simulink model "xPC_UDP"  (R2016a)
settings: Solver=ode3  StartTime=0.0  StopTime=inf  FixedStep=dt  RelTol=1e-3
InitFcn:
  | XPCUDP_DEPENDENCY
  | init_xPC_UDP
  | init_udp
undefined symbols (not defined in the file or in its folder): dt
libraries: etargetslib x2, xpcrtudplib x2, slrtlib x1, xpcobsoletelib x1, simulink x1
settings Model: Creator=Andrea  LastModifiedBy=garrison
settings SolverCC: EnableConcurrentExecution=on
settings DataIOCC: LimitDataPoints=on  SaveFormat=Array  SignalLoggingSaveFormat=ModelDataLogs
settings OptimizationCC: BlockReduction=off  OptimizeBlockIOStorage=off  BufferReuse=off  GlobalBufferReuse=off  ExpressionFolding=off  ExpressionDepthLimit=2147483647  LocalBlockOutputs=off  OptimizeModelRefInitCode=on
settings DebuggingCC: UnderspecifiedInitializationDetection=Classic  MergeDetectMultiDrivingBlocksExec=none  SolverPrmCheckMsg=warning  MultiTaskCondExecSysMsg=warning  MultiTaskRateTransMsg=warning  FcnCallInpInsideContextMsg=UseLocalSettings  StateNameClashWarn=warning
settings HardwareCC: ProdBitPerPointer=32  ProdLargestAtomicFloat=None  ProdWordSize=32  ProdLongLongMode=on  ProdHWDeviceType=Generic->32-bit x86 compatible
settings ModelReferenceCC: PropagateSignalLabelsOutOfModel=off
settings SFSimCC: SimParseCustomCode=off
settings RTWCC: SystemTargetFile=slrtert.tlc  TemplateMakefile=slrtert_default_tmf  Description=Simulink Real-Time (ERT)  RTWCompilerOptimization=on
settings CodeAppCC: CustomSymbolStrType=$N$R$M  InternalIdentifier=Classic
settings SimulinkRealTimeERTCC: TargetFcnLib=ansi_tfl_table_tmw.mat  GenFloatMathFcnCalls=NOT IN USE  TargetLangStandard=C89/C90 (ANSI)  CodeReplacementLibrary=XPC_BLAS  UtilityFuncGeneration=Auto  ERTMultiwordTypeDef=System defined  ERTMultiwordLength=256  MultiwordLength=2048  GenerateFullHeader=on  InferredTypesCompatibility=off  GenerateSampleERTMain=off  GenerateTestInterfaces=off  ModelReferenceCompliant=on  ParMdlRefBuildCompliant=on  CompOptLevelCompliant=on  ConcurrentExecutionCompliant=on  IncludeMdlTerminateFcn=on  GeneratePreprocessorConditionals=Disable all  CombineOutputUpdateFcns=off  CombineSignalStateStructs=off  SuppressErrorStatus=off  ERTFirstTimeCompliant=off  IncludeFileDelimiter=Auto  ERTCustomFileBanners=off  SupportAbsoluteTime=on  LogVarNameModifier=rt_  MatFileLogging=on  MultiInstanceERTCode=off  CodeInterfacePackaging=Nonreusable function  SupportNonFinite=on  SupportComplex=on  PurelyIntegerCode=off  SupportContinuousTime=on  SupportNonInlinedSFcns=on  SupportVariableSizeSignals=off  ParenthesesLevel=Nominal  CastingMode=Nominal  MATLABClassNameForMDSCustomization=xpcAperiodicCustomization  ModelStepFunctionPrototypeControlCompliant=off  CPPClassGenCompliant=off  AutosarCompliant=off  GRTInterface=on  GenerateAllocFcn=off  UseToolchainInfoCompliant=off  GenerateSharedConstants=on  ExtModeTransport=0  ExtModeStaticAlloc=off  ExtModeStaticAllocSize=1000000  ExtModeTesting=off  InlinedParameterPlacement=Hierarchical  TargetOS=BareBoardExample  MultiInstanceErrorCode=Error  RateGroupingCode=on  RootIOFormat=Individual arguments  RTWCAPIRootIO=off  EnableDataOwnership=off  ERTFilePackagingFormat=Modular  PreserveExpressionOrder=off  PreserveIfCondition=off  ConvertIfToSwitch=off  PreserveExternInFcnDecls=on  SuppressUnreachableDefaultCases=off  EnableSignedLeftShifts=on  EnableSignedRightShifts=on  IndentStyle=K&R  IndentSize=2  EnableUserReplacementTypes=off  MaxIdInt32=MAX_int32_T  MinIdInt32=MIN_int32_T  MaxIdUint32=MAX_uint32_T  MaxIdInt16=MAX_int16_T  MinIdInt16=MIN_int16_T  MaxIdUint16=MAX_uint16_T  MaxIdInt8=MAX_int8_T  MinIdInt8=MIN_int8_T  MaxIdUint8=MAX_uint8_T  BooleanTrueId=true  BooleanFalseId=false  MemSecPackage=--- None ---  MemSecDataConstants=Default  MemSecDataIO=Default  MemSecDataInternal=Default  MemSecDataParameters=Default  MemSecFuncInitTerm=Default  MemSecFuncExecute=Default  MemSecFuncSharedUtil=Default  GlobalDataDefinition=Auto  GlobalDataReference=Auto  GenerateASAP2=off  ERTSrcFileBannerTemplate=ert_code_template.cgt  ERTHdrFileBannerTemplate=ert_code_template.cgt  ERTDataSrcFileTemplate=ert_code_template.cgt  ERTDataHdrFileTemplate=ert_code_template.cgt  ERTCustomFileTemplate=example_file_process.tlc  SignalDisplayLevel=10  ParamTuneLevel=10  InitialValueSource=Model  RTWCAPISignals=off  RTWCAPIParams=on  RTWCAPIStates=off  RL32ModeModifier=Real-Time  ExtMode=on  ExtModeMexFile=ext_xpc  ExtModeIntrfLevel=Level2 - Open  ExtModeArmWhenConnect=off  RL32LogTETModifier=on  RL32LogBufSizeModifier=100000  xPCTaskExecutionProfile=off  xPCRL32EventNumber=5000  RL32IRQSourceModifier=Timer  xPCIRQSourceBoard=None/Other  xPCIOIRQSlot=-1  xpcObjCom=off  xPCGenerateASAP2=off  xPCGenerateXML=off  RL32ObjectName=tg  xPCisDownloadable=off  xPCisDefaultEnv=on  xPCisModelTimeout=on  xPCModelTimeoutSecs=5  xpcDblBuff=off  xPCLoadParamSetFile=off  xPCConcurrentTasks=off  xPCEnableSFAnimation=off
settings ConfigComp: CovModelRefEnable=Off

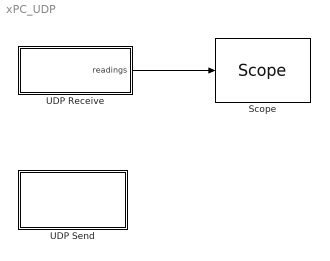
== system xPC_UDP ==
  "Scope " : slrtlib/Displays and Logging/Scope   scopeno=1  scopetype=Target  autostart=on  viewmode=Numerical  formatstr='%15.6f'  grid=on  ylimits=[0,0]  nosamples=250  noprepostsamples=0  interleave=1  triggermode=FreeRun  triggersignal=1  trigsignalfromport=off  triggerlevel=0.0  triggerslope=Either  triggerscope=1  triggersample=0  filename=data.dat  mode=Lazy  writesize=512  autorestart=off  dynamicfilemode=off  maxwritefilesize=512*1024^2
  UDP Receive : Subsystem  TreatAsAtomicUnit=on
      mask Display: %image(imread('trakSTAR.jpg'));
  UDP Send : Subsystem
  wires:
  UDP Receive/1(readings) -> "Scope "/1

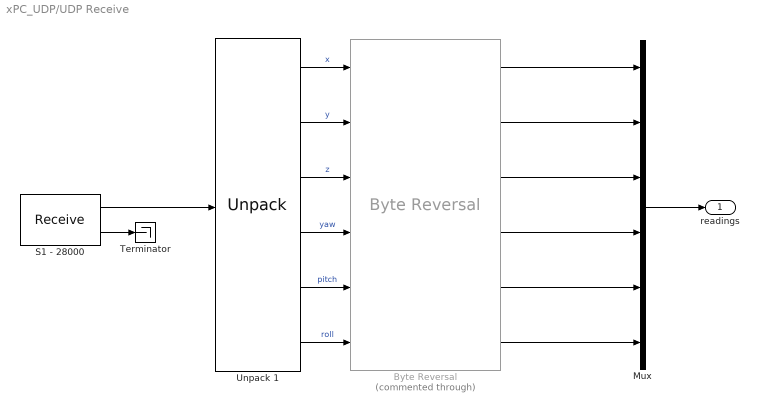
== system xPC_UDP/UDP Receive ==
  Byte Reversal : etargetslib/Byte Reversal  Commented=through  numInp=6
  Mux : Mux  Inputs=6
  S1 - 28000 : xpcrtudplib/Legacy UDP/Receive   ipAddress=0.0.0.0  ipPort=28000  width=48  vblLen=on  sampletime=dt_udp
  Terminator : Terminator
  Unpack 1 : xpcobsoletelib/Utilities/Unpack   dimensions={1,1,1,1,1,1}  datatypes={'double' 'double' 'double' 'double' 'double' 'double'}  byteAlign=1
  readings : Outport
  wires:
  S1 - 28000/1 -> Unpack 1/1
  S1 - 28000/2 -> Terminator/1
  Byte Reversal/1 -> Mux/1
  Byte Reversal/2 -> Mux/2
  Byte Reversal/3 -> Mux/3
  Byte Reversal/4 -> Mux/4
  Byte Reversal/5 -> Mux/5
  Byte Reversal/6 -> Mux/6
  Unpack 1/6 -> Byte Reversal/6  "roll"
  Unpack 1/5 -> Byte Reversal/5  "pitch"
  Unpack 1/4 -> Byte Reversal/4  "yaw"
  Unpack 1/3 -> Byte Reversal/3  "z"
  Unpack 1/2 -> Byte Reversal/2  "y"
  Unpack 1/1 -> Byte Reversal/1  "x"
  Mux/1 -> readings/1

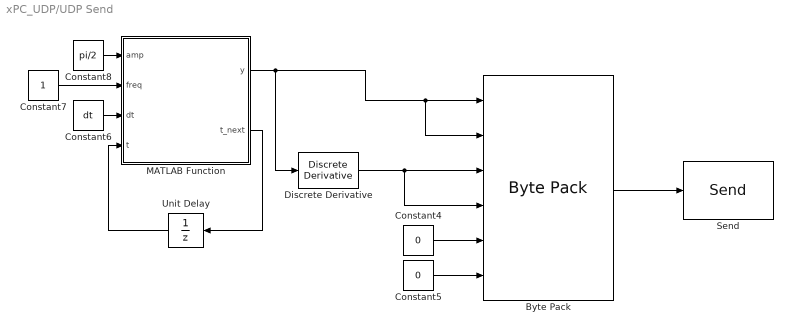
== system xPC_UDP/UDP Send ==
  Byte Pack : etargetslib/Byte Pack  datatypes={'double' 'double' 'double' 'double' 'double' 'double'}  byteAlign=1
  Constant4 : Constant  Value=0
  Constant5 : Constant  Value=0
  Constant6 : Constant  Value=dt
  Constant7 : Constant
  Constant8 : Constant  Value=pi/2
  Discrete Derivative : simulink/Discrete/Discrete Derivative  gainval=1  ICPrevScaledInput=0.0  OutMin=[]  OutMax=[]  OutDataType=fixdt(1, 16)  OutScaling=2^-10  DoSatur=off
  MATLAB Function : MATLAB Function  TreatAsAtomicUnit=on
  "Send " : xpcrtudplib/Legacy UDP/Send   ipAddress=192.168.1.30  ipPort=28001  localPort=-1  vblLen=off  sampletime=dt_udp
  Unit Delay : UnitDelay  SampleTime=-1
  wires:
  Byte Pack/1 -> "Send "/1
  Constant5/1 -> Byte Pack/6
  Discrete Derivative/1 -> Byte Pack/3, Byte Pack/4
  Constant4/1 -> Byte Pack/5
  MATLAB Function/1(y) -> Discrete Derivative/1, Byte Pack/2, Byte Pack/1
  MATLAB Function/2(t_next) -> Unit Delay/1
  Unit Delay/1 -> MATLAB Function/4(t)
  Constant6/1 -> MATLAB Function/3(dt)
  Constant7/1 -> MATLAB Function/2(freq)
  Constant8/1 -> MATLAB Function/1(amp)

== matlab function xPC_UDP/UDP Send/MATLAB Function ==
  data: amp input; freq input; dt input; y output; t input; t_next output
function [y,t_next] = fcn(amp,freq,dt,t)
%#codegen

y = amp*sin(2*pi*freq*t);
t_next = t + dt;
